simulink model "time_variance_test"  (R2024b)
settings: Solver=ode4  StartTime=0.0  StopTime=3  FixedStep=1e-3  RelTol=1e-3
settings Model: Creator=auralius  LastModifiedBy=auralius

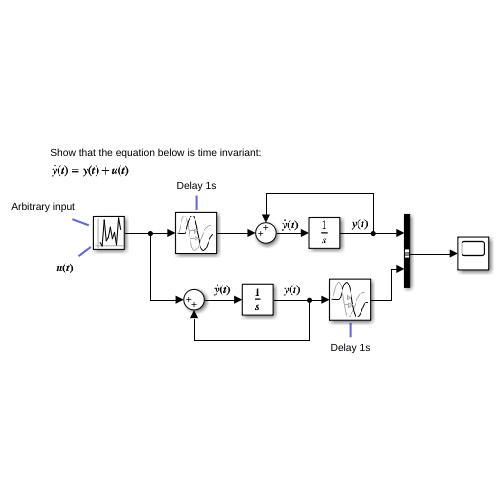
[thumbnail: Simulink's stored preview of the top-level diagram]
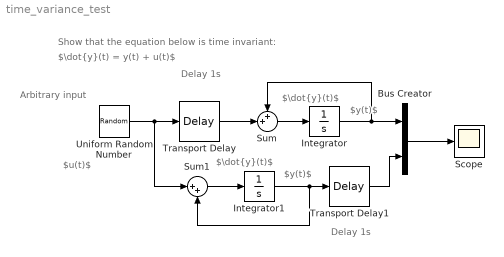
== system time_variance_test ==
  note: $\dot{y}(t)$
  note: $y(t)$
  note: $u(t)$
  note: Show that the equation below is time invariant:
  note: $\dot{y}(t) = y(t) + u(t)$
  note: Arbitrary input
  note: Delay 1s
  note: Delay 1s
  note: $y(t)$
  note: $\dot{y}(t)$
  Bus Creator : BusCreator  Inputs=2
  Integrator : Integrator
  Integrator1 : Integrator
  Scope : Scope
  Sum : Sum  Inputs=++|
  Sum1 : Sum  Inputs=|++
  Transport Delay : TransportDelay
  Transport Delay1 : TransportDelay
  Uniform Random Number : UniformRandomNumber
  wires:
  Bus Creator/1 -> Scope/1
  Transport Delay1/1 -> Bus Creator/2
  Integrator/1 -> Bus Creator/1, Sum/1
  Integrator1/1 -> Transport Delay1/1, Sum1/2
  Sum1/1 -> Integrator1/1
  Uniform Random Number/1 -> Transport Delay/1, Sum1/1
  Transport Delay/1 -> Sum/2
  Sum/1 -> Integrator/1
